simulink model "Simu_Kinematics_Dynamics_Model_2014"  (R2015a)
settings: Solver=ode45  SolverMode=SingleTasking  StartTime=0.0  StopTime=1000.0  RelTol=1e-3
InitFcn:
  | addpath('../parameters/')
  | aircraft_parameters
  | simulation_parameters
undefined symbols (not defined in the file or in its folder): drawAircraft, plotmavstatevariables
libraries: simulink x6
settings Model: CovMetricSettings=dwe  CovHtmlReporting=off  covSaveCumulativeToWorkspaceVar=off  CovSaveSingleToWorkspaceVar=off  CovExternalEMLEnable=on  Creator=h1huang  LastModifiedBy=User
settings DataIOCC: LimitDataPoints=off  SaveFormat=StructureWithTime  ReturnWorkspaceOutputs=on
settings DebuggingCC: SFUnexpectedBacktrackingDiag=error  SFNoUnconditionalDefaultTransitionDiag=error
settings HardwareCC: ProdBitPerPointer=64  ProdLargestAtomicFloat=Float  ProdIntDivRoundTo=Zero  ProdEndianess=LittleEndian  ProdHWDeviceType=Specified
settings ModelReferenceCC: PropagateSignalLabelsOutOfModel=on
settings SFSimCC: SimUseLocalCustomCode=on
settings RTWCC: RTWUseLocalCustomCode=on
settings GRTTargetCC: TargetLangStandard=C99 (ISO)

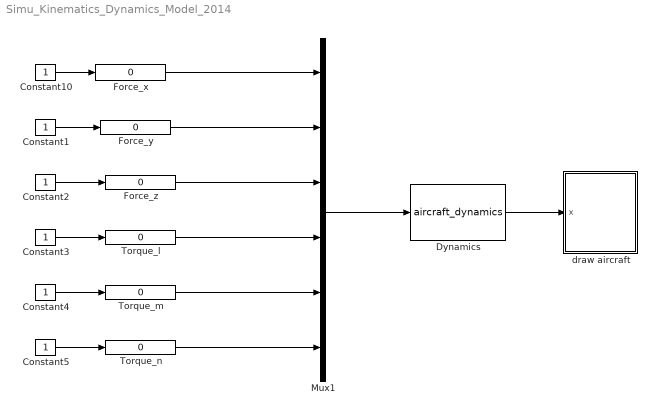
== system Simu_Kinematics_Dynamics_Model_2014 ==
  Constant{1..5,10} (6 alike) : Constant
  Dynamics : S-Function  FunctionName=aircraft_dynamics  Parameters=UAV
  Force_x : simulink/Math Operations/Slider Gain  low=-1  gain=0  high=1
  Force_y : simulink/Math Operations/Slider Gain  low=-1  gain=0  high=1
  Force_z : simulink/Math Operations/Slider Gain  low=-1  gain=0  high=1
  Mux1 : Mux  Inputs=6
  Torque_l : simulink/Math Operations/Slider Gain  low=-0.1  gain=0  high=0.1
  Torque_m : simulink/Math Operations/Slider Gain  low=-0.1  gain=0  high=0.1
  "Torque_n " : simulink/Math Operations/Slider Gain  low=-0.1  gain=0  high=0.1
  draw aircraft : Subsystem
      mask Display: image(imread('../chap2/tv.jpg'))
  wires:
  Mux1/1 -> Dynamics/1
  Constant3/1 -> Torque_l/1
  Force_x/1 -> Mux1/1
  Torque_m/1 -> Mux1/5
  Constant4/1 -> Torque_m/1
  Constant1/1 -> Force_y/1
  Force_z/1 -> Mux1/3
  Constant2/1 -> Force_z/1
  Torque_l/1 -> Mux1/4
  Force_y/1 -> Mux1/2
  "Torque_n "/1 -> Mux1/6
  Dynamics/1 -> draw aircraft/1(x)
  Constant10/1 -> Force_x/1
  Constant5/1 -> "Torque_n "/1

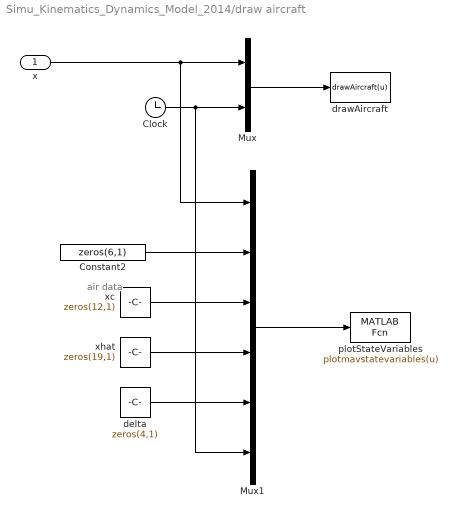
== system Simu_Kinematics_Dynamics_Model_2014/draw aircraft ==
  note: air data
  x : Inport
  Clock : Clock
  Constant2 : Constant  Value=zeros(6,1)
  Mux : Mux  Inputs=2
  Mux1 : Mux  Inputs=6
  delta : Constant  Value=zeros(4,1)
  drawAircraft : MATLABFcn  MATLABFcn=drawAircraft(u)  OutputDimensions=0  SampleTime=0.1
  plotStateVariables : MATLABFcn  MATLABFcn=plotmavstatevariables(u)  OutputDimensions=0  SampleTime=0.1
  xc : Constant  Value=zeros(12,1)
  xhat : Constant  Value=zeros(19,1)
  wires:
  Mux/1 -> drawAircraft/1
  x/1 -> Mux/1, Mux1/1
  Clock/1 -> Mux/2, Mux1/6
  Mux1/1 -> plotStateVariables/1
  xhat/1 -> Mux1/4
  xc/1 -> Mux1/3
  delta/1 -> Mux1/5
  Constant2/1 -> Mux1/2
